simulink model "Turntable_close_step_2017b"  (R2018b)
settings: Solver=ode3  StartTime=0.0  StopTime=40  FixedStep=0.0005  RelTol=1e-3
InitFcn:
  | para_test
values from neighbouring files (symbols this model uses):
  denominator = cell2mat(controller.Denominator)    [sweep_close.m]
  gain = b0    (= 23249.4996924)    [para_test.m]
  J = 1.076    [sweep_close.m]
  Kps = 1.077250780790937e+02    (= 107.725078079)    [sweep_close.m]
  Kt = 24.812626200641272    (= 24.8126262006)    [sweep_close.m]
  Kv = 0.12    [sweep_close.m]
  L = 0.733240176511722    (= 0.733240176512)    [sweep_close.m]
  numerator = cell2mat(controller.Numerator)    [sweep_close.m]
  r = 80.116666666666666667    (= 80.1166666667)    [sweep_close.m]
settings Model: Creator=Vera  LastModifiedBy=57531
settings OptimizationCC: LifeSpan=inf
settings DebuggingCC: SFExecutionAtInitializationDiag=none
settings SFSimCC: SimUseLocalCustomCode=off
settings RTWCC: RTWUseLocalCustomCode=off
settings CodeAppCC: StateflowObjectComments=on

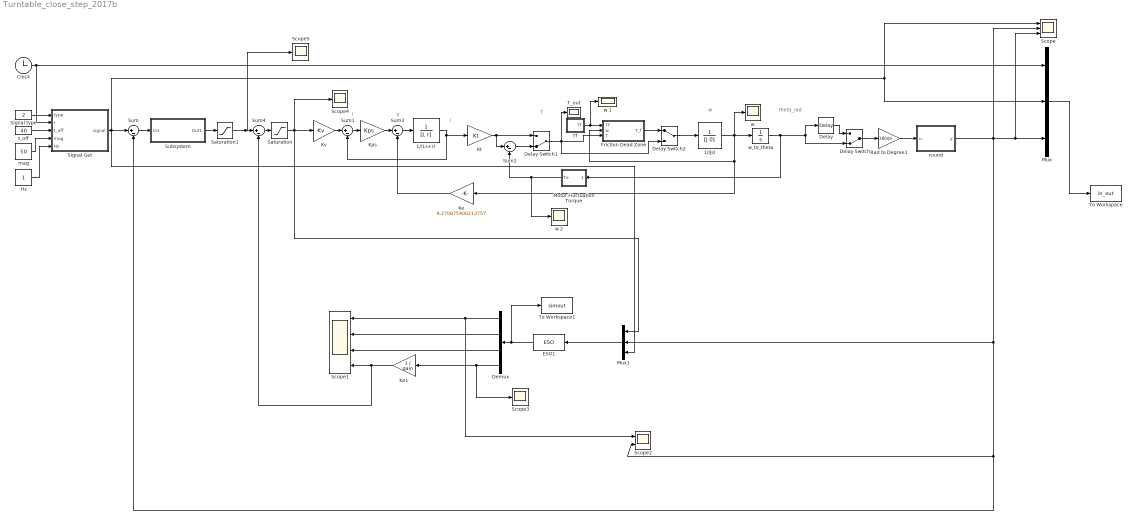
== system Turntable_close_step_2017b ==
  note: i
  note: w
  note: V
  note: i
  note: T
  note: theta_rad
  " Delay Switch" : ManualSwitch  CurrentSetting=0
  " Delay Switch1" : ManualSwitch  CurrentSetting=0
  " Delay Switch2" : ManualSwitch
  1/(Js) : TransferFcn  Denominator=[J 0]
  1/(Ls+r) : TransferFcn  Denominator=[L r]
  Clock : Clock
  Delay : TransportDelay  DelayTime=0.003763900000000
  Demux : Demux
  ESO1 : S-Function  FunctionName=ESO  SFunctionDeploymentMode=off  EnableBusSupport=off
  Friction Dead Zone : MATLAB Function  TreatAsAtomicUnit=on
  Hz : Constant
  Ke : Gain  Gain=8.270875400213757
  Ke1 : Gain  Gain=1 / gain
  Kps : Gain  Gain=Kps
  Kt : Gain  Gain=Kt
  Kv : Gain  Gain=Kv
  Motor Fluctuation Torque : Subsystem
  Mux : Mux  Inputs=3
  Mux1 : Mux  Inputs=3
  Rad to Degree1 : Gain  Gain=180/pi
  Saturation : Saturate  UpperLimit=10  LowerLimit=-10
  Saturation1 : Saturate  UpperLimit=10  LowerLimit=-10
  Scope : Scope  NumInputPorts=3
  Scope1 : Scope  NumInputPorts=4
  Scope2 : Scope  NumInputPorts=2
  Scope3 : Scope
  Scope4 : Scope
  Scope5 : Scope
  Signal Get : MATLAB Function  TreatAsAtomicUnit=on
  Signal type : Constant  Value=2
  Subsystem : Subsystem
  Sum{,1..4} (5 alike) : Sum  Inputs=|+-
  T_out : Scope
  Tf : Subsystem
  To Workspace : ToWorkspace  VariableName=in_out  SampleTime=-1
  To Workspace1 : ToWorkspace  VariableName=simout  SaveFormat=Timeseries  SampleTime=-1
  mag : Constant  Value=50
  round : MATLAB Function  TreatAsAtomicUnit=on
  t_off : Constant  Value=40
  "w " : Scope
  w 1 : Scope
  w 2 : Scope
  w_to_theta : Integrator
  wires:
  t_off/1 -> Signal Get/3(t_off)
  Clock/1 -> Mux/1, Signal Get/2(t)
  mag/1 -> Signal Get/4(mag)
  Hz/1 -> Signal Get/5(Hz)
  Kv/1 -> Sum1/1
  Motor Fluctuation Torque/1(Te) -> w 2/1, Sum2/2
  Tf/1(Tf) -> w 1/1, Friction Dead Zone/1(Tf)
  1/(Ls+r)/1 -> Sum1/2, Kt/1
  Sum3/1 -> 1/(Ls+r)/1
  Delay/1 -> " Delay Switch"/1
  w_to_theta/1 -> Delay/1, " Delay Switch"/2, Motor Fluctuation Torque/1(theta)
  " Delay Switch"/1 -> Rad to Degree1/1
  1/(Js)/1 -> "w "/1, w_to_theta/1, Friction Dead Zone/2(w), Ke/1
  Ke/1 -> Sum3/2
  Sum1/1 -> Kps/1
  Kt/1 -> " Delay Switch1"/1, Sum2/1
  Kps/1 -> Sum3/1
  Mux/1 -> To Workspace/1
  Signal type/1 -> Signal Get/1(type)
  Signal Get/1(signal) -> Mux1/3, Sum/1, Mux/2, Scope/1
  " Delay Switch2"/1 -> 1/(Js)/1
  Friction Dead Zone/1(T_f) -> " Delay Switch2"/1
  Sum2/1 -> " Delay Switch1"/2
  " Delay Switch1"/1 -> " Delay Switch2"/2, Friction Dead Zone/3(T), T_out/1
  Sum/1 -> Subsystem/1(In1)
  ESO1/1 -> To Workspace1/1, Demux/1
  Mux1/1 -> ESO1/1
  Demux/2 -> Scope1/2
  Demux/4 -> Scope3/1, Ke1/1
  Demux/3 -> Scope1/3
  Demux/1 -> Scope2/1, Scope1/1
  Subsystem/1(Out1) -> Saturation1/1
  Saturation/1 -> Kv/1, Mux1/1, Scope4/1
  Sum4/1 -> Saturation/1
  Ke1/1 -> Sum4/2, Scope1/4
  Rad to Degree1/1 -> round/1(u)
  Saturation1/1 -> Scope5/1, Sum4/1
  round/1(y) -> Scope2/2, Sum/2, Mux1/2, Scope/2, Scope/3, Mux/3

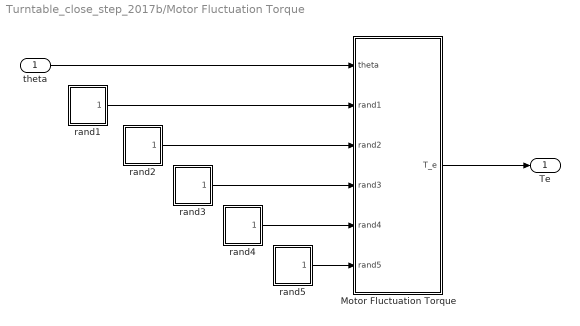
== system Turntable_close_step_2017b/Motor Fluctuation Torque ==
  theta : Inport
  Motor Fluctuation Torque : MATLAB Function  TreatAsAtomicUnit=on
  rand1 : Subsystem
  rand2 : Subsystem
  rand3 : Subsystem
  rand4 : Subsystem
  rand5 : Subsystem
  Te : Outport
  wires:
  theta/1 -> Motor Fluctuation Torque/1(theta)
  rand1/1(rand1) -> Motor Fluctuation Torque/2(rand1)
  rand2/1(rand2) -> Motor Fluctuation Torque/3(rand2)
  rand3/1(rand3) -> Motor Fluctuation Torque/4(rand3)
  rand4/1(rand4) -> Motor Fluctuation Torque/5(rand4)
  rand5/1(rand5) -> Motor Fluctuation Torque/6(rand5)
  Motor Fluctuation Torque/1(T_e) -> Te/1

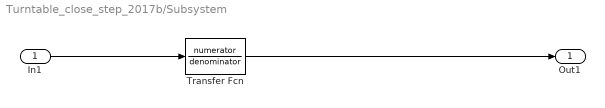
== system Turntable_close_step_2017b/Subsystem ==
  In1 : Inport
  Transfer Fcn : TransferFcn  Numerator=numerator  Denominator=denominator
  Out1 : Outport
  wires:
  Transfer Fcn/1 -> Out1/1
  In1/1 -> Transfer Fcn/1

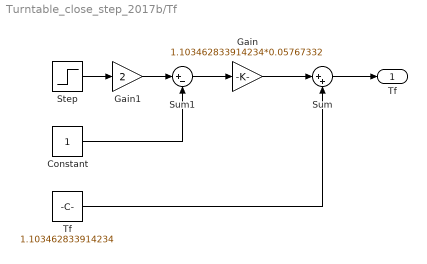
== system Turntable_close_step_2017b/Tf ==
  Constant : Constant
  Gain : Gain  Gain=1.103462833914234*0.05767332
  Gain1 : Gain  Gain=2
  Step : Step  Time=0  After=rand  SampleTime=0
  Sum : Sum  Inputs=|++
  Sum1 : Sum  Inputs=|+-
  "Tf " : Constant  Value=1.103462833914234  VectorParams1D=off
  Tf : Outport
  wires:
  Gain/1 -> Sum/1
  "Tf "/1 -> Sum/2
  Sum/1 -> Tf/1
  Step/1 -> Gain1/1
  Gain1/1 -> Sum1/1
  Constant/1 -> Sum1/2
  Sum1/1 -> Gain/1

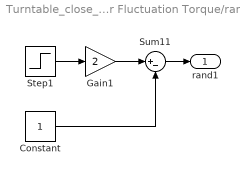
== system Turntable_close_step_2017b/Motor Fluctuation Torque/rand1 ==
  Constant : Constant
  Gain1 : Gain  Gain=2
  Step1 : Step  Time=0  After=rand  SampleTime=0
  Sum11 : Sum  Inputs=|+-
  rand1 : Outport
  wires:
  Step1/1 -> Gain1/1
  Gain1/1 -> Sum11/1
  Constant/1 -> Sum11/2
  Sum11/1 -> rand1/1

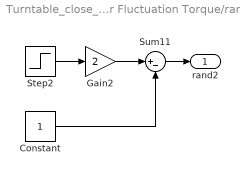
== system Turntable_close_step_2017b/Motor Fluctuation Torque/rand2 ==
  Constant : Constant
  Gain2 : Gain  Gain=2
  Step2 : Step  Time=0  After=rand  SampleTime=0
  Sum11 : Sum  Inputs=|+-
  rand2 : Outport
  wires:
  Step2/1 -> Gain2/1
  Gain2/1 -> Sum11/1
  Constant/1 -> Sum11/2
  Sum11/1 -> rand2/1

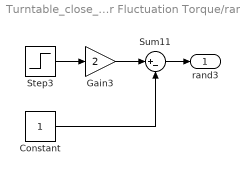
== system Turntable_close_step_2017b/Motor Fluctuation Torque/rand3 ==
  Constant : Constant
  Gain3 : Gain  Gain=2
  Step3 : Step  Time=0  After=rand  SampleTime=0
  Sum11 : Sum  Inputs=|+-
  rand3 : Outport
  wires:
  Sum11/1 -> rand3/1
  Constant/1 -> Sum11/2
  Gain3/1 -> Sum11/1
  Step3/1 -> Gain3/1

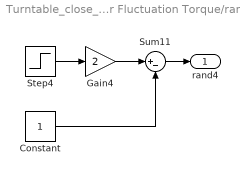
== system Turntable_close_step_2017b/Motor Fluctuation Torque/rand4 ==
  Constant : Constant
  Gain4 : Gain  Gain=2
  Step4 : Step  Time=0  After=rand  SampleTime=0
  Sum11 : Sum  Inputs=|+-
  rand4 : Outport
  wires:
  Step4/1 -> Gain4/1
  Gain4/1 -> Sum11/1
  Constant/1 -> Sum11/2
  Sum11/1 -> rand4/1

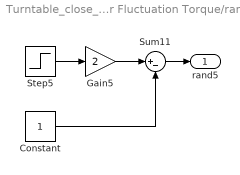
== system Turntable_close_step_2017b/Motor Fluctuation Torque/rand5 ==
  Constant : Constant
  Gain5 : Gain  Gain=2
  Step5 : Step  Time=0  After=rand  SampleTime=0
  Sum11 : Sum  Inputs=|+-
  rand5 : Outport
  wires:
  Sum11/1 -> rand5/1
  Constant/1 -> Sum11/2
  Gain5/1 -> Sum11/1
  Step5/1 -> Gain5/1

== matlab function Turntable_close_step_2017b/Signal Get ==
  data: type input; t input; t_off input; mag input; signal output; Hz input
function signal = fcn(type, t, t_off, mag, Hz)
signal = 0;
switch type
    case 1
        w = 2 * pi * Hz;
        if((t >= 0) && (t < 1))
            signal = t * mag * sin(w * t);
        elseif((t >= 1) && (t < t_off - 1))
            signal = mag * sin(w * t);
        elseif((t >= (t_off - 1)) && (t < t_off))
            signal = -mag * (t - t_off) * sin(w * t);
        else
            signal = 0;
        end
    case 2
        if t < 10
            signal = t * mag / 10;
        elseif t >= 10 && t < (t_off - 10)
            signal = mag;
        elseif t >= (t_off - 10) && t < t_off
            signal = (t_off - t) * mag / 10;
        else
            signal = 0;
        end
        
end

== matlab function Turntable_close_step_2017b/Friction Dead Zone ==
  data: Tf input; w input; T input; T_f output
function T_f = fcn(Tf,w,T)
if w==0
    if abs(T)<abs(Tf)
        T_f = 0;
    else
        T_f=sign(T)*(abs(T)-Tf);
    end
elseif w*T<0
    T_f=sign(T)*(abs(T)+Tf);
else 
        if abs(T)<abs(Tf)
            T_f = -sign(w)*(Tf-abs(T));
        else
            T_f=sign(T)*(abs(T)-Tf);
        end

end
end

== matlab function Turntable_close_step_2017b/round ==
  data: u input; y output
function y = fcn(u)
y = round(u * 10000) / 10000;

== matlab function Turntable_close_step_2017b/Motor Fluctuation Torque/Motor Fluctuation Torque ==
  data: T_e output; theta input; rand1 input; rand2 input; rand3 input; rand4 input; rand5 input
function T_e = fcn(theta,rand1,rand2,rand3,rand4,rand5)
T_p =0.432273269433135*(1+rand1*0.012015015613962)*cos(theta*7 +(48.13841636+0.050850865438431)*pi/180);
T_2p=0.035501355062786*(1+rand2*0.032198449030114)*cos(theta*14+(30.38979755+0.101746126073106)*pi/180);
T_4p=0.018930935537422*(1+rand3*0.028225982587057)*cos(theta*28+(285.7823597+0.203848223609672)*pi/180);
T_6p=0.012218243879728*(1+rand4*0.058230694793342)*cos(theta*42+(152.9148096+0.306666606518932)*pi/180);
T_45=0.009203318745614*(1+rand5*0.098213466988815)*cos(theta*45+(279.6898495+0.328827530537396)*pi/180);

T_e=1 * (T_p + T_2p + T_4p + T_6p + T_45);
end
